simulink model "Delay2"  (R2020a)
settings: Solver=VariableStepAuto  StartTime=0.0  StopTime=10.0  RelTol=1e-3
settings Model: Creator=bzhan  LastModifiedBy=bzhan

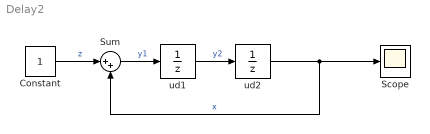
== system Delay2 ==
  Constant : Constant
  Scope : Scope
  Sum : Sum  Inputs=|++
  ud1 : UnitDelay  HasFrameUpgradeWarning=on
  ud2 : UnitDelay  HasFrameUpgradeWarning=on
  wires:
  Constant/1 -> Sum/1  "z"
  ud2/1 -> Scope/1, Sum/2  "x"
  Sum/1 -> ud1/1  "y1"
  ud1/1 -> ud2/1  "y2"
